simulink model "ModelForSlidesFeb"  (R2023a)
settings: Solver=VariableStepAuto  StartTime=0  StopTime=1000  FixedStep=0.01  RelTol=1e-3
model workspace (MAT data in the model file):
  finalint = 0
  firstWarning = 1
  originalScenarioChecksum = '114339432DE22364D47BB28FC96DC10C'
undefined symbols (not defined in the file): Acceleration, ActorID, AngularVelocity, curvature, DefaultGear, Defined, DEND_B, DEND_S, DEND_T, direction, DiscIntNeverNeededParam, driving, Ego, gradbp, L, Lane, LF, LR, m, matlabshared, MAX_BRAKE, MAX_STEER, MAX_TORQUE, maxNumActors, MCAR, MIN_BRAKE, MIN_STEER, MIN_TORQUE, n, NUMD_B, NUMD_S, NUMD_T, Pitch, Pose, Position, psi_o, R, Roll, RRdamp, SceneInfo, session, sigbuilder_block, STEER_RATIO, stopSign_ID, Tdead, thetaRefs, TL_ID, TrackWidth, ts, Ts, User, Vdead, Velocity, WB, X_o, xRef2s, Y_o, Yaw, yRef2s
libraries: drivingscenarioandsensors x13, roadrunnerscenario x11, simulink x8, simulink_extras x5, drivingvehiclecontroller x2, trackingutilitieslib x2, robotalgslib x1, mpcadaslib x1, slpidlib x1, drivinglib x1, autolibshared x1, vehdynlibviscommon x1
(part 4 of 4)

== matlab function ModelForSlidesFeb/Subsystem/Function-Call Subsystem/MATLAB Function2 ==
  data: EgoPosition input; MIOPos input; curvature input; MIOVel input; V_i input; xd output; yd output; laneL input; laneR input; V_desired input; LCinProgress output
function [xd,yd,LCinProgress] = traj(EgoPosition,MIOPos,curvature,MIOVel, V_i, laneL, laneR, V_desired)
Vx_i =0;Vx_f=0;Vy_i=0;Vy_f=0;Ax_i=0;Ax_f=0;Ay_i=0;Ay_f=0;T_i=0;T_f=0;V_f=0;A_f=0;x_set=0;y_set=0;theta4=0;

P = zeros(6,6);
% xq = zeros(1,size(RefPath,1)); yq = zeros(1,size(RefPath,2));
EgoPosition(1,2)=-EgoPosition(1,2)
x_init= EgoPosition(1,1)+0.5; y_init = EgoPosition(1,2)-0.8;
% xq = RefPath(:,1)'; 
% yq = RefPath(:,2)';
num_foc_t = 98;
V_max= V_desired; ad_n=0; vd_n=MIOVel; wd_n=vd_n*curvature;
lane_width = 3.6 * (laneL-laneR); % +1 if left of current lane and -1 if right of current lane
xd = zeros(num_foc_t+1,1); 
yd = zeros(num_foc_t+1,1);
xf =0; 
yf = 0;

    %xf = [EgoPosition(1,1)+ MIOPos(1) ]; yf = [ EgoPosition(1,2)+ MIOPos(2) + lane_width];  
    xf = [EgoPosition(1,1)+ 40 ]; yf = [ EgoPosition(1,2)+ 1.1*lane_width]; % 80
    V_f = V_max;
    W_f = V_f*curvature;
    A_f = 0;

    %dist2crash = sqrt((x_init-MIOPos(1))^2+(y_init-MIOPos(2))^2);
    %dist2crash = 40;
    %T_f = abs(dist2crash/(MIOVel-V_i));
    T_f = 3;
    P = [1, T_i, T_i^2, T_i^3, T_i^4, T_i^5;
         0, 1, 2*T_i, 3*T_i^2, 4*T_i^3, 5*T_i^4;
         0, 0, 2, 6*T_i, 12*T_i^2, 20*T_i^3;
         1, T_f, T_f^2, T_f^3, T_f^4, T_f^5;
         0, 1, 2*T_f, 3*T_f^2, 4*T_f^3, 5*T_f^4;
         0, 0, 2, 6*T_f, 12*T_f^2, 20*T_f^3];

%     mtang4 = (yq(1,index+2)-yq(1,index+1))/(xq(1,index+2)-xq(1,index+1));

    Vx_i = vd_n*cos(theta4); 
    Vy_i = vd_n*sin(theta4); 
    Ax_i = ad_n*cos(theta4)-vd_n*sin(theta4)*wd_n; 
    Ay_i = ad_n*sin(theta4)+vd_n*cos(theta4)*wd_n;

%     if(xq(index+2)-xq(index+1)<0)
%         theta_4 = pi + atan(mtang4);
%     else
%         theta_4 = atan(mtang4);
%     end

    theta_4 =0;
    Vx_f = V_f*cos(theta_4); % curvature angle
    Vy_f = V_f*sin(theta_4);
    Ax_f = A_f*cos(theta_4)-V_f*sin(theta_4)*W_f;
    Ay_f = A_f*sin(theta_4)+V_f*cos(theta_4)*W_f;

    g1 = [x_init; Vx_i; Ax_i; xf; Vx_f; Ax_f];
    g2 = [y_init; Vy_i; Ay_i; yf; Vy_f; Ay_f];

    a_coeff = P\g1;
    b_coeff = P\g2;
    
    td = T_i;
    scatter(x_init,y_init,'go')
    hold on; 
    scatter(xf,yf,'ro')
    hold on;
    
    for f = 1:(num_foc_t+1)
        xd(f,1) = [1,td,td^2,td^3,td^4,td^5]*a_coeff 
        yd(f,1) = [1,td,td^2,td^3,td^4,td^5]*b_coeff
        td = td + (T_f - T_i)/num_foc_t;
        scatter(xd(f,1),yd(f,1),'y.');
    end

LCinProgress = 1;

% hold on;
end

== matlab function ModelForSlidesFeb/Controllers/MATLAB Function2 ==
  data: v input; RefVelCmd output; curvature input
function RefVelCmd = fcn(v,curvature)

    if abs(curvature) >= 0 && abs(curvature) <= 2e-2
        RefVelCmd = v;
    else
        r = 1/abs(curvature);
        RefVelCmd = min(v,sqrt(9.81*r*.2));
    end

== matlab function ModelForSlidesFeb/Vehicle Dynamics/Info2ActorState/MATLAB Function1 ==
  data: Xdot input; Velocity output; Ydot input; Zdot input
function Velocity = fcn(Xdot, Ydot, Zdot)

Velocity = [Xdot Ydot, Zdot];

== matlab function ModelForSlidesFeb/MATLAB Function ==
  data: ttc output; dist output; left output; right output; LL_avail output; RL_avail output; tend2stay output; ego input; act input; LaneBounds input; RoadSpeed input; ego_vel output; stay output; LL_Change output; RL_Change output; y_lane output; LCinProgress input
function [ttc,dist,left,right,LL_avail,RL_avail,tend2stay,ego_vel,stay,LL_Change,RL_Change,y_lane] = fcn(ego,act,LaneBounds,RoadSpeed, LCinProgress)                       


%% Major tasks to look into

% Check the performance while transitioning into another lane 
% Lane change output when the ego on extreme lanes.
% Develop code to handle lane changes on road curvatures
% Integrate with the trajectory generation and check the perfomance
% Convert the code to ego vehicle coordinates


%%
%define some parameters
r_c = 20; %range considered to MIOs
t_min =  2;

num_actors = length(act.Actors);
%num_lanes = length(LaneBounds.LaneBoundaries)-1;


%% Using sensor data 
% TracksNum = Tracking.NumTracks;
% 
% 
% for t = 1:TracksNum
%     ObjectID(t) = Tracking.Tracks(t).ObjectClassID;
%     TrackPos(:,t) = Tracking.Tracks(t).State(1:2:5);
%     TrackVel(:,t) = Tracking.Tracks(t).State(2:2:6);

%% ego position and  velocity magnitude
ego_pos = ego.Position;
ego_vel = ego.Velocity(1);  % velocity

%ttc: (array) : agent.relative position / abs(relative velocity)
ttc = zeros(1,num_actors);
left = zeros(1,num_actors);
right = zeros(1,num_actors);

dist =  zeros(1,num_actors);
tend2stay=1;

%%
y_lane = zeros(1,length(LaneBounds.LaneBoundaries))

for l=1:length(y_lane)
    y_lane(l)=LaneBounds.LaneBoundaries(l).Coordinates(end,2)
end

%%
for i= 1:num_actors

    % Grab actor positions and velocities
    actor_pos = act.Actors(i).Position;   
    actor_vel = act.Actors(i).Velocity(1);  % x-component velocity

    %relative velocity of the agent
    rel_vel = actor_vel - ego_vel;


    %% Check if the actor is within a r_c range. If it is out of range, pass lane change as '1' automatically.

   dist(i) = norm([actor_pos(1) actor_pos(2)]-[ego_pos(1) ego_pos(2)]);
        
    if dist(i) > r_c
        left(i)=1;
        right(i)=1;
        continue
    end

    %% Check if the actor is in the same lane as that of ego

    % If the actor and ego are in the same lane, it is considered a lead/following vehicle in the same lane and by defualt, the lane change flag is 1.

    if (actor_pos(2)< (ego_pos(2)+0.5) && actor_pos(2) > (ego_pos(2)-0.5))
        if (rel_vel < 0 && ego_vel < (RoadSpeed+5) && actor_pos(1) > ego_pos(1) )
            left(i) =1;
            right(i)=1;
            tend2stay=0;        % we need to incorporate too slow condition even when the relative velocity is greater than 0.

        elseif (rel_vel < 0 && ego_vel < (RoadSpeed+5) && actor_pos(1) < ego_pos(1) )
            left(i) =1;
            right(i)=1;
            tend2stay=1;
        end

        continue
    end

    
    %% calculate ttc for the rest of the vehicles


    ttc(i) = (actor_pos(1)-ego_pos(1))/abs(rel_vel);

    % checking conditions for other surrounding actors

    % all actors on the left lane of the ego vehicle
%%
    if actor_pos(2)-ego_pos(2) > 0  

        if and(rel_vel>0, ttc(i) > t_min)  % target vehicles on the front of ego vehicle (any lane)
    
            left(i)=1; 
            right(i)=1;
    
        elseif (ttc(i)<0 && rel_vel<0 && abs(ttc(i)) > t_min)    % target vehicle on the back of ego vehicle (ttc<0) (any lane)
            left(i) =1;
            right(i)=1;
    
        else 
            left(i) =0;
            right(i)=1;
    
        end

    % all actors on the right lane of the ego vehicle

    elseif actor_pos(2)-ego_pos(2) < 0
         
        if and(rel_vel>0, ttc(i) > t_min)  % target vehicles on the front of ego vehicle (any lane)
    
            left(i)=1;
            right(i)=1;
    
        elseif (ttc(i)<0 && rel_vel<0 && abs(ttc(i)) > t_min)    % target vehicle on the back of ego vehicle (ttc<0) (any lane)
            left(i) =1;
            right(i)=1;
    
        else 
            left(i) =1;
            right(i)=0;
    
        end
    end
%%

end

%% check if the vehicle is in the extreme end lanes

    if ego_pos(2)<y_lane(1) && ego_pos(2)>y_lane(2)

        LL=0; RL=1;
    elseif ego_pos(2) > y_lane(end) && ego_pos(2) < y_lane(end-1)
        RL=0; LL=1;
    else 

        RL=1;LL=1;
    end

%%
LL_avail = all(left) %&& LL;

RL_avail = all(right) %&& RL               %&& ~lcLeft ; this can be decided later 


%% final commands

stay = tend2stay || ~(tend2stay || LL_avail || RL_avail);
LL_Change =  ~tend2stay && LL_avail ;

RL_Change =  ~tend2stay && RL_avail && ~LL_Change ;
LCFlag = ~stay;
if LCFlag && LCinProgress
    LCFlag = false;
    stay = ~LCFlag;
end

%% 






end

== matlab function ModelForSlidesFeb/Vehicle Dynamics/Info2ActorState/MATLAB Function2 ==
  data: aX input; Acceleration output; aY input; aZ input
function Acceleration = fcn(aX, aY, aZ)

Acceleration = [aX aY, aZ];

== matlab function ModelForSlidesFeb/Vehicle Dynamics/Info2ActorState/MATLAB Function3 ==
  data: phiDot input; AngularVelocity output; thetaDot input; psiDot input
function AngularVelocity = fcn(phiDot, thetaDot, psiDot)

AngularVelocity = [phiDot thetaDot, psiDot];

== stateflow chart ModelForSlidesFeb/Vehicle Dynamics/VehicleDynamics/engine-steer-brake dynamics/GearSelection1 ==
  state Park
    CurrGear = 0;
  state Reverse
    CurrGear = -1;
  state drive
    CurrGear = 1;
  (default) -> (junction 12)
  (junction 12) -> Reverse [order 3] : [DefaultGear == -1]
  (junction 12) -> drive [order 2] : [DefaultGear == 1]
  (junction 12) -> Park [order 1] : [DefaultGear == 0]
  (junction 12) -> Park [order 4] : %fallback to park
  drive -> Park [order 2] : [gear_cmd == 0 && allowShift(vc,Tbrake)]
  Park -> Reverse [order 2] : [gear_cmd == -1 && allowShift(vc,Tbrake)]
  Park -> drive [order 1] : [gear_cmd == 1 && allowShift(vc,Tbrake)]
  Reverse -> Park [order 2] : [gear_cmd == 0 && allowShift(vc,Tbrake)]
  drive -> Reverse [order 1] : [gear_cmd == -1 && allowShift(vc,Tbrake)]
  Reverse -> drive [order 1] : [gear_cmd == 1 && allowShift(vc,Tbrake)]
  data: Tdead parameter; Vdead parameter; vel function_input; brakeT function_input; allow function_output; CurrGear output; Tbrake input; vc input; gear_cmd input; DefaultGear parameter
  function allow = allowShift(vel, brakeT):
    | function allow = allowShift(vel, brakeT)
    | allow = (abs(vel) <= Vdead) && (abs(brakeT)>Tdead);
    | end

== matlab function ModelForSlidesFeb/Vehicle Dynamics/VehicleDynamics/engine-steer-brake dynamics/compute net torque ==
  data: gear input; Tnet output; Tengine input; Tbrake input; vc input
function Tnet  = net_torque(gear,Tengine,Tbrake,vc)

%  --set engine torque based on current gear selection

if (gear == 0)
    %  --vehicle is in PARK, so force engine torque to zero
    Tengine = 0;
end

Tnet = Tengine + Tbrake*tanh(5*vc);

end

== matlab function ModelForSlidesFeb/Vehicle Dynamics/VehicleDynamics/engine-steer-brake dynamics/gear selection state machine ==
  data: gear output; gear_cmd input; vc input; Tbrake input; Tdead input; Vdead input
function gear = gear_change_FSM(gear_cmd,vc,Tbrake,Tdead,Vdead)

persistent GEAR

%  The vehicle gear can take on one of the following enumerated values:
%  -1 = REVERSE
%   0 = PARK
%   1 = DRIVE

%  --initialize the local persistent variables

if isempty(GEAR)
    %  --default gear at startup is PARK
    %  Note:  Change this to 1 if you want car to initialize in DRIVE
    GEAR = 0;
end


%  --evaluate the gear change finite state machine

switch GEAR
    case 0  % vehicle is in PARK
        if (gear_cmd == 1)
            %  --check to see if we can shift to DRIVE
            if ((abs(vc) <= Vdead) && (abs(Tbrake) > Tdead))
                %  --shift to DRIVE
                GEAR = 1;
            end
            
        elseif (gear_cmd == 2)
            %  --check to see if we can shift to REVERSE
            if ((abs(vc) <= Vdead) && (abs(Tbrake) > Tdead))
                %  --shift to REVERSE
                GEAR = 2;
            end
        end
        
    case 1  % vehicle is in DRIVE
        if (gear_cmd == 0)
            %  --check to see if we can shift to PARK
            if ((abs(vc) <= Vdead) && (abs(Tbrake) > Tdead))
                %  --shift to PARK
                GEAR = 0;
            end
            
        elseif (gear_cmd == 2)
            %  --check to see if we can shift to REVERSE
            if ((abs(vc) <= Vdead) && (abs(Tbrake) > Tdead))
                %  --shift to REVERSE
                GEAR = 2;
            end
        end
        
    case -1  % vehicle is in REVERSE
        if (gear_cmd == 0)
            %  --check to see if we can shift to PARK
            if ((abs(vc) <= Vdead) && (abs(Tbrake) > Tdead))
                %  --shift to PARK
                GEAR = 0;
            end
            
        elseif (gear_cmd == 1)
            %  --check to see if we can shift to DRIVE
            if ((abs(vc) <= Vdead) && (abs(Tbrake) > Tdead))
                %  --shift to DRIVE
                GEAR = 1;
            end
        end
        
    otherwise  %  --should never be here
        if (vc > Vdead)
            %  --moving forward, so must be in DRIVE
            GEAR = 1;
        elseif (vc < -Vdead)
            %  --moving backward, so must be in REVERSE
            GEAR = 2;
        else
            %  --vehicle stoppped, so must be in PARK
            GEAR = 0;
        end

end


%  --output the current actual gear setting

gear = GEAR;

return

== matlab function ModelForSlidesFeb/Behavioural Planner/MATLAB Function3 ==
  data: Dest input; D2D output; CurrentPose input
function D2D = fcn(Dest, CurrentPose)

% CurrentPose(2) = -CurrentPose(2);

% For RoadRunner
Dest = [Dest(2) Dest(1)]; 
CurrentPose = [CurrentPose(2) CurrentPose(1)];
D2D = norm(Dest - CurrentPose(1:2));

% D2D=sqrt((CurrentPose(1)-Dest(1,1))^2+(CurrentPose(2)-Dest(1,2))^2);
end

== stateflow chart ModelForSlidesFeb/Behavioural Planner/Chart ==
  settings: updateMethod=DISCRETE  sampleTime=Ts
  state Stationary
    en,du:
    VelCmd = 0;
    CurrentVelCmd = VelCmd;
    Navi = 0;
    Trans = 0;
    StopSim = 0;
    Tgap = 1;
    HoldBrake = 1;
    Braking = 0;
  state Navigation
    state RailCrossing
      state Stop
        en:
        VelCmd = 0;
        Braking = 1;
        CurrentVelCmd = VelCmd;
      state Approaching
        en:
        Braking = 1;
        Tgap = 0;
        Trans = 0;
      state Transition
        en:
        Tgap = 1;
        Trans = 1;
        Braking = 0;
        VelCmd = SceneSpeed;
        CurrentVelCmd = VelCmd;
      state ExitScene
        en:
        ExitFlag = 1;
      (default) -> Navigation.RailCrossing.Approaching
      Navigation.RailCrossing.Approaching -> Navigation.RailCrossing.Stop [order 1] : [D2S <= 6 && (RRCross == 1 || ObjectDist <= TransDist)]
      Navigation.RailCrossing.Transition -> Navigation.RailCrossing.Approaching [order 2] : [ObjectDist <= TransDist]
      Navigation.RailCrossing.Approaching -> Navigation.RailCrossing.Transition [order 3] : [RRCross == 0 && ObjectDist > TransDist && D2S <= 6]
      Navigation.RailCrossing.Stop -> Navigation.RailCrossing.Transition : [RRCross == 0 && ObjectDist > TransDist]
      Navigation.RailCrossing.Approaching -> Navigation.RailCrossing.ExitScene [order 2] : [SceneID ~= 10]
      Navigation.RailCrossing.Transition -> Navigation.RailCrossing.ExitScene [order 1] : [SceneID == 0]
    state RoundAbout
      state Approaching
        en:
        Braking = 1;
        Trans = 0;
        Tgap = 0;
      state Stop
        en:
        VelCmd = 0;
        Braking = 1;
        CurrentVelCmd = VelCmd;
      state ExitScene
        en:
        ExitFlag = 1;
      state Transition
        en:
        Tgap = 1;
        Trans = 1;
        Braking = 0;
        VelCmd = SceneSpeed;
        CurrentVelCmd = VelCmd;
      (default) -> Navigation.RoundAbout.Approaching
      Navigation.RoundAbout.Approaching -> Navigation.RoundAbout.Stop [order 1] : [D2S <= 6]
      Navigation.RoundAbout.Stop -> Navigation.RoundAbout.Transition : [Clear2Go == 1]
      Navigation.RoundAbout.Approaching -> Navigation.RoundAbout.ExitScene [order 2] : [SceneID ~= 9]
      Navigation.RoundAbout.Transition -> Navigation.RoundAbout.ExitScene : [SceneID == 0]
    state DestCheck
      en,du:
      % dest reached?
      (default) -> (junction 47)
      (junction 47) -> (junction 48) [order 1] : [D2D < 2]
      (junction 47) -> (junction 49) [order 2] : {DestReached = 0;}
      (junction 48) -> (junction 50) : {DestReached = 1;}
      (junction 50) -> (junction 49) : {StopSim = 1;}
      (junction 49) -> (junction 51)
    state TrafficLight [commented out]
      note: Yellow light duration is 1s
      state Stop [commented out]
        en:
        Braking = 1;
        VelCmd = 0;
        CurrentVelCmd = VelCmd;
      state Approaching [commented out]
        en:
        Tgap = 0;
        Trans = 0;
        T2S = 0;
        %if TLstate(1,4) == 1
        Braking = 1;
        %else
        % ACC = 0;
        %end
      state DecisionOnYellow [commented out]
        en:
        T2S = D2S/EgoSpeed;
      state Transition [commented out]
        en:
        Trans = 1;
        Braking = 0;
        Tgap = 1;
        VelCmd = SceneSpeed;
        CurrentVelCmd = VelCmd;
      state ExitScene [commented out]
        en:
        ExitFlag = 1;
      DecisionOnYellow -> Navigation.TrafficLight.Approaching [commented out] : [T2S > 1.2]
      (default) -> Navigation.TrafficLight.Approaching [commented out]
      Navigation.TrafficLight.Approaching -> Navigation.TrafficLight.Stop [commented out] : [D2S <= 6]
      Navigation.TrafficLight.Stop -> Navigation.TrafficLight.Transition [commented out] : [TLstate(1,4) == 3 && ObjectDist > TransDist]
      Navigation.TrafficLight.Transition -> Navigation.TrafficLight.Approaching [commented out] : [TLstate(1,4) == 1  || ObjectDist < TransDist]
      Navigation.TrafficLight.Approaching -> Navigation.TrafficLight.Transition [commented out] : [TLstate(1,4) == 3 && ObjectDist > TransDist]
      Navigation.TrafficLight.Approaching -> Navigation.TrafficLight.ExitScene [commented out] : [SceneID ~= 8]
      Navigation.TrafficLight.Transition -> DecisionOnYellow [commented out] : [TLstate(1,4) == 2]
      DecisionOnYellow -> Navigation.TrafficLight.Transition [commented out] : [T2S <= 1.2]
      Navigation.TrafficLight.Transition -> Navigation.TrafficLight.ExitScene [commented out] : [SceneID == 0]
    state Drive
      en :
      HoldBrake = 0;
      VelCmd = RoadSpeed;
      CurrentVelCmd = VelCmd;
      ExitFlag = 0;
    state Go
      en:
      VelCmd = RoadSpeed;
      CurrentVelCmd = VelCmd;
      Trans = 0;
      ExitFlag = 0;
      Braking = 0;
      HoldBrake = 1;
    state StopSign
      state StoptSign4way
        state CheckInt
          du:
          % stopped?
          % ss priority?
        state CheckSS
          % stopped?
          % ss priority?
        state Transition
          en:
          % stay here while trans?!
          % while ~crossedLimitLine of TargetLane
          Trans = 1;
          Braking = 0;
          Tgap = 1;
          VelCmd = SceneSpeed;
          CurrentVelCmd = VelCmd;
        state ExitScene
          en:
          ExitFlag = 1;
        (default) -> Navigation.StopSign.StoptSign4way.CheckSS
        Navigation.StopSign.StoptSign4way.CheckSS -> Navigation.StopSign.StoptSign4way.CheckInt : [EgoSpeed < VelStop]
        Navigation.StopSign.StoptSign4way.CheckInt -> Navigation.StopSign.StoptSign4way.Transition : [egoSSPriority == 1 && Clear2Go == 1]
        Navigation.StopSign.StoptSign4way.Transition -> Navigation.StopSign.StoptSign4way.ExitScene : [SceneID == 0 && after(2,sec)]
      state SStype
        state Approaching
          en:
          %VelCmd = ApproachingSpeed;
          Braking = 1;
          Trans = 0;
          Tgap = 0;
        state Stop
          en:
          VelCmd = 0;
          Braking = 1;
          CurrentVelCmd = VelCmd;
        Navigation.StopSign.SStype.Stop -> 410 [order 1] : [numSS == 4]
        (default) -> Navigation.StopSign.SStype.Approaching
        Navigation.StopSign.SStype.Approaching -> Navigation.StopSign.SStype.Stop : [D2S <= 15]
        Navigation.StopSign.SStype.Stop -> 414 [order 2] : [numSS == 2]
      state StopSign2way
        state CheckInt
          en:
          VelCmd = 0;
          HoldBrake = 1;
          CurrentVelCmd = VelCmd;
        state CheckSS
          % stopped?
          % ss priority?
        state Transition1
          en:
          % stay here while trans?!
          % while ~crossedLimitLine of TargetLane
          Trans = 1;
          Braking = 0;
          HoldBrake = 0;
          Tgap = 1;
          VelCmd = SceneSpeed;
          CurrentVelCmd = VelCmd;
        state ExitScene1
          en:
          ExitFlag = 1;
        (default) -> Navigation.StopSign.StopSign2way.CheckSS
        Navigation.StopSign.StopSign2way.CheckSS -> Navigation.StopSign.StopSign2way.CheckInt : [EgoSpeed < VelStop]
        Navigation.StopSign.StopSign2way.CheckInt -> Transition1 : [egoSSPriority == 1 && ToAClearance == 1 && after(1,sec)]
        Transition1 -> Navigation.StopSign.StopSign2way.CheckInt [order 2] : [ToAClearance == 0]
        Transition1 -> ExitScene1 [order 1] : [SceneID == 0 && egoExit == 1]
      (default) -> SStype
      416 -> StoptSign4way
      411 -> StopSign2way
    Go -> RailCrossing [order 2] : [SceneID == 10]
    Drive -> RailCrossing [order 1] : [SceneID == 10]
    RailCrossing -> Go : [ExitFlag == 1]
    Go -> RoundAbout [order 3] : [SceneID == 9]
    Drive -> RoundAbout [order 2] : [SceneID == 9]
    RoundAbout -> Go : [ExitFlag == 1]
    (default) -> DestCheck
    Drive -> TrafficLight [commented out] : [SceneID == 8]
    DestCheck -> Drive : [DestReached == 0]
    Go -> TrafficLight [commented out] : [SceneID == 8]
    Drive -> DestCheck [order 4] : [D2D < 2]
    TrafficLight -> Go [commented out] : [ExitFlag == 1]
    Drive -> StopSign [order 3] : [SceneID == 7]
    StopSign -> Go : [ExitFlag == 1]
    Go -> DestCheck [order 1] : [SceneID == 0]
    Go -> StopSign [order 4] : [SceneID == 7]
  (default) -> Stationary
  Stationary -> Navigation : [Navigate == 1]
  Navigation -> Stationary : [Navigate == 0 || DestReached == 1]
  data: TLstate input; numSS input; egoExit input; ToAClearance input; TransDist input; ApproachingSpeed input; EgoSpeed input; ObjectDist input; SceneSpeed input; SDist input; RRCross input; D2S input; DestReached local; Navigate input; ExitFlag local; D2D input; Clear2Go input; RoadSpeed input; CurrentVelCmd local; Navi local; VelCmd output; HoldBrake output; SceneID input; Tgap output; Trans output; StopSim output; Braking output; T2S local; VelStop input; egoSSPriority input

== matlab function ModelForSlidesFeb/Subsystem/Function-Call Subsystem/MATLAB Function1 ==
  data: EgoPosition input; MIOPos input; curvature input; MIOVel input; V_i input; xd output; yd output; laneL input; laneR input; V_desired input; LCinProgress output
function [xd,yd,LCinProgress] = traj(EgoPosition,MIOPos,curvature,MIOVel, V_i, laneL, laneR, V_desired)
Vx_i =0;Vx_f=0;Vy_i=0;Vy_f=0;Ax_i=0;Ax_f=0;Ay_i=0;Ay_f=0;T_i=0;T_f=0;V_f=0;A_f=0;x_set=0;y_set=0;theta4=0;

P = zeros(6,6);
% xq = zeros(1,size(RefPath,1)); yq = zeros(1,size(RefPath,2));
EgoPosition(1,2)=-EgoPosition(1,2);
x_init= EgoPosition(1,1)+2; y_init = EgoPosition(1,2)-2;
% xq = RefPath(:,1)'; 
% yq = RefPath(:,2)';
num_foc_t = 98;
V_max= V_desired; ad_n=0; vd_n=MIOVel; wd_n=vd_n*curvature;
lane_width = 3.6 * (laneL-laneR); % +1 if left of current lane and -1 if right of current lane(rahul flipped)
xd = zeros(num_foc_t+1,1); 
yd = zeros(num_foc_t+1,1);
xf =0; 
yf = 0;

    %xf = [EgoPosition(1,1)+ MIOPos(1) ]; yf = [ EgoPosition(1,2)+ MIOPos(2) + lane_width];  
    xf = [EgoPosition(1,1)+ 20 ]; yf = [EgoPosition(1,2)+ lane_width]; % 80
    V_f = V_max;
    W_f = V_f*curvature;
    A_f = 0;

    %dist2crash = sqrt((x_init-MIOPos(1))^2+(y_init-MIOPos(2))^2);
    %dist2crash = 40;
    %T_f = abs(dist2crash/(MIOVel-V_i));
    T_f = 3;
    P = [1, T_i, T_i^2, T_i^3, T_i^4, T_i^5;
         0, 1, 2*T_i, 3*T_i^2, 4*T_i^3, 5*T_i^4;
         0, 0, 2, 6*T_i, 12*T_i^2, 20*T_i^3;
         1, T_f, T_f^2, T_f^3, T_f^4, T_f^5;
         0, 1, 2*T_f, 3*T_f^2, 4*T_f^3, 5*T_f^4;
         0, 0, 2, 6*T_f, 12*T_f^2, 20*T_f^3];

%     mtang4 = (yq(1,index+2)-yq(1,index+1))/(xq(1,index+2)-xq(1,index+1));

    Vx_i = vd_n*cos(theta4); 
    Vy_i = vd_n*sin(theta4); 
    Ax_i = ad_n*cos(theta4)-vd_n*sin(theta4)*wd_n; 
    Ay_i = ad_n*sin(theta4)+vd_n*cos(theta4)*wd_n;

%     if(xq(index+2)-xq(index+1)<0)
%         theta_4 = pi + atan(mtang4);
%     else
%         theta_4 = atan(mtang4);
%     end

    theta_4 =0;
    Vx_f = V_f*cos(theta_4); % curvature angle
    Vy_f = V_f*sin(theta_4);
    Ax_f = A_f*cos(theta_4)-V_f*sin(theta_4)*W_f;
    Ay_f = A_f*sin(theta_4)+V_f*cos(theta_4)*W_f;

    g1 = [x_init; Vx_i; Ax_i; xf; Vx_f; Ax_f];
    g2 = [y_init; Vy_i; Ay_i; yf; Vy_f; Ay_f];

    a_coeff = P\g1;
    b_coeff = P\g2;
    
    td = T_i;
    scatter(x_init,y_init,'go')
    hold on; 
    scatter(xf,yf,'ro')
    hold on;
    
    for f = 1:(num_foc_t+1)
        xd(f,1) = [1,td,td^2,td^3,td^4,td^5]*a_coeff 
        yd(f,1) = [1,td,td^2,td^3,td^4,td^5]*b_coeff
        td = td + (T_f - T_i)/num_foc_t;
        scatter(xd(f,1),yd(f,1),'y.');
    end

LCinProgress = 1;

% hold on;
end

== matlab function ModelForSlidesFeb/Behavioural Planner/StopSignPriority ==
  settings: updateMethod=DISCRETE
  data: ToAClearance output; SDist input; D2S input; ObjTracks input; egoSSPriority output; SceneTracks input; egoPose input; egoSpeed input; numSS output; VelStop input; WB input; d output; flag input; flag output; midpoint input; midpoint output; egoExit output; egoEnter input; egoEnter output; egoExitang output; egoExitdist output
function [ToAClearance, egoSSPriority, numSS, d, flag, midpoint, egoExit, egoEnter, egoExitang, egoExitdist]  = StopSignPriority(SDist, D2S, ObjTracks, SceneTracks, egoPose, egoSpeed, VelStop, WB, flag, midpoint, egoEnter)
% calculate covariance matrix outside, input to this block is modified with final, unique detections
egoPose = [-egoPose(2) egoPose(1) 90+egoPose(3)];
persistent SSPriority C1x C2y C3x C4y
% find stop signs + one of 2way or 4way or T-junction

% find number of signs (until we reach 0 valued columns)
numSS = 0;
for j = 1:length(SceneTracks(1,:))
    if any(SceneTracks(:,j))
        numSS = numSS + 1;
    end
end

% find number of cars
numCars = 0;
for j = 1:length(ObjTracks(1,:))
    if any(ObjTracks(:,j))
        numCars = numCars + 1;
    end
end


egoSSPriority = 1;
ToAClearance = 1;
actorExitang = 0;
ToAThreshold = 5;
% tempPriority = zeros(numCars+1,1);
d = zeros(10, 5); % distance, velocity, time, location (wrt ego), exit (leaving ints)
Objang = zeros(10, 1);
% priorityTable = zeros(numCars+1, 5);
egoExitang = egoPose(3) - atan2d(midpoint(2)-egoPose(2),midpoint(1)-egoPose(1)); % 0 deg = straight , + = right
egoExitdist = sqrt((midpoint(2)-egoPose(2))^2+(midpoint(1)-egoPose(1))^2);

if abs(egoExitang) >= 135 && egoExitdist >= 10 && egoEnter == 1
    d(1,5) = 1; % ego left the ints
    egoEnter = 0;
    flag = 0;
elseif abs(egoExitang) >= 135 && egoExitdist <= 20 && egoExitdist >= 10
    d(1,5) = 1;
end

egoExit = d(1,5);


if (D2S <= SDist || egoEnter == 1) && egoExitdist >= 9

    % [~, index] = min(abs(SceneTracks(1,:)'));
    if numSS > 0

        Vmd = [-egoSpeed*sind(egoPose(3)), egoSpeed*cosd(egoPose(3))];
        rot = [cosd(egoPose(3)) -sind(egoPose(3)); sind(egoPose(3)) cosd(egoPose(3))];
        

        % intersection region
        if flag == 0
            C1x = min(SceneTracks(1, 1:numSS)) - (WB + 3);
            C2y = min(SceneTracks(3, 1:numSS)) - (WB + 3);
            C3x = max(SceneTracks(1, 1:numSS)) + (WB + 3);
            C4y = max(SceneTracks(3, 1:numSS)) + (WB + 3);
            C1 = rot*[C1x; C2y] + egoPose(1:2)';
            C2 = rot*[C3x; C4y] + egoPose(1:2)';
            midpoint = (C1+C2)./2;
            
            % C1x = min(SceneTracks(1, 1:numSS)) - (WB + 3);
            % C2y = min(SceneTracks(3, 1:numSS)) - (WB + 3);
            % C3x = max(SceneTracks(1, 1:numSS)) + (WB + 3);
            % C4y = max(SceneTracks(3, 1:numSS)) + (WB + 3);
            % midpoint = [2*egoPose(1)-C4y-C2y; 2*egoPose(2)+C1x+C3x]./2;
        %   scatter(-SceneTracks(3,:)+egoPose(1),SceneTracks(1,:)+egoPose(2),'blue','filled')   
            % scatter(midpoint(1), midpoint(2), 'blue', 'filled')
            % rectangle('Position',[egoPose(1)-C4y egoPose(2)+C1x abs(C4y-C2y) abs(C3x-C1x)])
            flag = C1x;
        end

        midpoint_ego = rot'*(midpoint - egoPose(1:2)');
        
        % loop through num of cars (j)
    
        d(1,1) = sqrt((midpoint(1) - egoPose(1))^2 + (midpoint(2) - egoPose(2))^2);
        d(1,2) = egoSpeed;
        d(1,3) = d(1,1)/d(1,2);     %add ego TOA
        d(1,4) = 4; % 4 is the location of the ego vehicle itself
        
        % if d(1,1) <= 3
        %     ToAThreshold = 2;
        % else
        %     ToAThreshold = 6;
        % end

        if d(1,1) <= flag
            egoEnter = 1;
        end

    
        % loop through signs (vectorized)
        % if smallest dist 
        % d(:,3) -> TOA = v/dist
    
        if numCars > 0
            for k = 1:numCars
                d(k+1,1) = sqrt((midpoint_ego(2)-ObjTracks(3,k))^2+(midpoint_ego(1)-ObjTracks(1,k))^2); %sqrt((midpoint(1) - (-ObjTracks(3,k)+egoPose(1)))^2 + (midpoint(2) - (ObjTracks(1,k)+egoPose(2)))^2); 
                d(k+1,2) = sqrt((Vmd(1) - ObjTracks(2,k))^2 + (Vmd(2) - ObjTracks(4,k))^2);
                d(k+1,3) = d(k+1,1)/d(k+1,2); % TOA of other cars
                Objang(k) = atan2d(ObjTracks(1,k), -ObjTracks(3,k));
                                
                % Identify cars location (direction) wrt ego
                if Objang(k) <= 60
                    d(k+1,4) = 1; % 1 = E, 2 = N, 3 = W
                elseif Objang(k) > 60  && Objang(k) < 120
                    d(k+1,4) = 2; % 1 = E, 2 = N, 3 = W
                elseif Objang(k) >= 120
                    d(k+1,4) = 3; % 1 = E, 2 = N, 3 = W
                end

                % Identifying leaving cars
                
                % ActorHeading = atan2d(ObjTracks(2,k) - Vmd(1), -ObjTracks(4,k) - Vmd(2));
                ActorHeading = atan2d(ObjTracks(2,k), ObjTracks(4,k));
                actorExitTheta = ActorHeading - atan2d(midpoint_ego(1)-ObjTracks(1,k),midpoint_ego(2)-ObjTracks(3,k));
                if actorExitTheta > 180
                    actorExitang = actorExitTheta - 360;
                else
                    actorExitang = actorExitTheta;
                end
                %actorExitdist = sqrt((midpoint_ego(2)-ObjTracks(3,k))^2+(midpoint_ego(1)-ObjTracks(1,k))^2);
                

                if abs(actorExitang) >= 135 && d(k+1,1) >= 10 
                    d(k+1,5) = 1; % left the ints
                else
                    d(k+1,5) = 0; % did not leave
                end

    
            end
    
            if numSS == 4 
                % Assign priorities based on rank TOA #1, before vehicle stops
                % d1 = d(d(:,1)~=0,:);
                [car, SSPriority] = sort(d(d(:,1)~=0 & d(:,5)==0));
                % priorityTable(:, 1:2) = [car, priority];
        
                tempPriority = find(SSPriority == 1); % ego SS priority
                if ~isempty(tempPriority)
                    egoSSPriority = tempPriority(1);
                end
            
            elseif numSS >= 1 && numSS < 4
                [car, SSPriority] = sort(d((d(:,4)==2 | d(:,4)==4) & d(:,5)==0));
                tempPriority = find(SSPriority == 1); % ego SS priority
                if ~isempty(tempPriority)
                    egoSSPriority = tempPriority(1);              
                end
                ToAClearance = double(all(d(d(:,1)~=0 & d(:,5)==0 & d(:,4)~=4,3) > ToAThreshold));
                
            end
    
        end
    end
    
    
    
    
    % if egoSpeed <= VelStop
    %     if SSPriority ~= 1
    %         % for all vehicles with higher priority
    %         % provide indicator signals to identify conflicts
    %         % check indicator signs/conflicts and update priority based on that
    %         % code to define leavingScene for other vehicles:
    %         % update priority table
    % 
    %     end
    % end
    
    
    
    

% elseif egoExit == 0
    

end

== matlab function ModelForSlidesFeb/Behavioural Planner/MATLAB Function1 ==
  data: EgoLength input; TransDist output; IntDist input
function TransDist = IntersectionClearanceDist(EgoLength,IntDist)

TransDist = IntDist + EgoLength;

== matlab function ModelForSlidesFeb/Subsystem/Turns LC in prog off ==
  data: u input; y output
function y = fcn(u)

persistent counter;
persistent input_high;

if isempty(counter)
    counter = 0;
end

if isempty(input_high)
    input_high = false;
end

if u ~= 0
    input_high = true;
end

if input_high && counter < 100
    y = u;
    counter = counter + 1;
else
    y = 0;
end

== matlab function ModelForSlidesFeb/Environment & Data/Roadrunner Port/ENU to NWD/MATLAB Function ==
  data: traj input; destination_traj output; last_idx output; Initial_traj output
function [destination_traj,last_idx,Initial_traj] = DestinationPoint(traj)

last_idx = 1;

for i=1:length(traj)
    if norm(traj(i,1:2)) == 0
        last_idx = i-1;
        break
    end
end

destination_traj = traj(last_idx,1:2);
Initial_traj = traj(1,1:2);

end

== matlab function ModelForSlidesFeb/Environment & Data/Roadrunner Port/ENU to NWD/MATLAB Function1 ==
  data: traj input; trajectory_way output
function trajectory_way = fcn(traj)

last_idx = 1;

for i=1:length(traj)
    if norm(traj(i,1:2)) == 0
        last_idx = i-1;
        break
    end
end

trajectory_way = zeros(150,2);

for j = 1:last_idx
    trajectory_way(j,:) = traj(j,1:2);
end


for k = (last_idx+1):100
    trajectory_way(k,:) = trajectory_way(last_idx,:);
end

== matlab function ModelForSlidesFeb/Environment & Data/Roadrunner Port/Initiaal State/Initialize State/Calculate Initial States/Calculate Initial States ==
  data: egoRuntime input; egoInitialState output Bus: BusVehicleInfo
function egoInitialState = getInitialState(egoRuntime)
%getInitialState calculates initial conditions of the vehicle

% Calculate velocity
velocity = norm(egoRuntime.ActorRuntime.Velocity,2);
% Get Transformation matrix
transformationMatrix = egoRuntime.ActorRuntime.Pose;
% Get pose information
x = transformationMatrix(1,4);
y = transformationMatrix(2,4);
yaw = atan2d(-transformationMatrix(1,2), ...
            transformationMatrix(1,1));
% Pack the initial states
egoInitialState = struct('CurrPose', [y, -x, yaw], ...
    'CurrVelocity', velocity, ...
    'CurrYawRate', 0, ...
    'CurrSteer',0, ...
    'Direction',1);

== matlab function ModelForSlidesFeb/Environment & Data/Roadrunner Port/MATLAB Function ==
  data: ActorsIn input; EgoVeh input; EgoRefActors output Bus: BusWorldToVehicleActors
function EgoRefActors  = GlobaltoEgoRefConv(ActorsIn,EgoVeh)
%ActorsOut = Simulink.Bus;
ActorsOut = ActorsIn;
numActors = length(ActorsIn.Actors);
for k = 1:numActors
    actorOut = driving.scenario.targetsToEgo(ActorsIn.Actors(k),EgoVeh);
    ActorsOut.Actors(k).ActorID             = actorOut.ActorID;
    ActorsOut.Actors(k).Position            = actorOut.Position;
    ActorsOut.Actors(k).Velocity            = actorOut.Velocity;
    ActorsOut.Actors(k).Roll                = actorOut.Roll;
    ActorsOut.Actors(k).Pitch               = actorOut.Pitch;
    ActorsOut.Actors(k).Yaw                 = actorOut.Yaw;
    ActorsOut.Actors(k).AngularVelocity    = actorOut.AngularVelocity;
end
EgoRefActors = ActorsOut;
end

== matlab function ModelForSlidesFeb/Subsystem/PathPlanner/MATLAB Function3 ==
  settings: updateMethod=DISCRETE
  data: out output; check output; Xref input; Yref input; xd input; yd input; LC input; current_pos input; d2f input; dcheck output
function [out,check,dcheck]  = PathPlanning(Xref, Yref, xd, yd, LC, current_pos, d2f)

persistent output_matrix
persistent lc_triggered

if isempty(lc_triggered)
lc_triggered = false;
end

%lc_triggered=0;
%if isempty(hold_output)
  %  hold_output = false;
%end


if isempty(output_matrix)
    output_matrix = [Xref(:), Yref(:)];
    out = [Xref(:), Yref(:)];
else
    out = output_matrix;
end

if LC && ~isempty(xd) && ~isempty(yd)
    output_matrix = [xd(:), yd(:)];
    lc_triggered=true;
       
end

check=lc_triggered;
dcheck=output_matrix;
%out=output_matrix;

if lc_triggered && d2f < 5 %&& ~isempty(output_matrix) %&& ~hold_output
    %Yout = Yref(:);
    if current_pos > 0
        Xout = Xref(:);
        Yout = Yref + 3.6;
    else
        Xout = Xref(:);
        Yout = Yref;
    end
    output_matrix = [Xout, Yout];
    out=output_matrix;
    lc_triggered=false;
    %hold_output = true;
end

out=output_matrix;




%if ~LC && ~isempty(output_matrix) && lc_triggered
    %hold_output = false;
    %lc_triggered=false;
%end

end

== matlab function ModelForSlidesFeb/Environment & Data/Roadrunner Port/MATLAB Function1 ==
  data: u input; long_out output; lat_out output; z_out output; out output; final_x output; final_y output
function [long_out, lat_out, z_out, out, final_x, final_y]  = fcn(u)
out = zeros(500, 3);
long = zeros(500, 1);
lat = zeros(500, 1);
long = u(:, 2);
lat = u(:,1);

for i = 1:500
    if long(i) == 0 && lat(i) == 0
        long(i) = long(i-1); 
        lat(i) = lat(i-1);
    end
end
final_x = lat(end);
final_y = long(end);
out(:,1) = lat;
out(:,2) = long;
out(:,3) = u(:, 3);

lat_out = out(:,1);
long_out = out(:, 2);
z_out =  out(:, 3);

== matlab function ModelForSlidesFeb/Environment & Data/Roadrunner Port/Pack Actor Pose/Pose Generation ==
  data: pose input; currPose output
function currPose = generatePose(pose)

yaw = deg2rad(pose(3));
rotm = eul2rotm([yaw 0 0]);

currPose = [[rotm [pose(1:2) 0]']; [0 0 0 1]];
% currPose = [[rotm [pose(1:2) 235]']; [0 0 0 1]];

== matlab function ModelForSlidesFeb/Environment & Data/Roadrunner Port/Pack Actor Pose/Velocity XYZ Components ==
  data: yaw input size=1; velocity output size=[1 3]; speed input size=1
function velocity = computeVelocity(yaw, speed)

% Output velocity vector (x,y,z)
velocity = speed * [-sind(yaw) cosd(yaw) 0];

== matlab function ModelForSlidesFeb/Environment & Data/Sensors & Perception/Tracking/MATLAB Function ==
  data: u input; y output; y1 output
function [y,y1] = fcn(u)
TracksNum = u.NumTracks;
y = zeros(20,1);
for k = 1:TracksNum
    y(k) = u.Tracks(k).ObjectAttributes.TargetIndex;
end
y1 = u.Tracks(1).ObjectAttributes.TargetIndex;

== matlab function ModelForSlidesFeb/Vehicle Dynamics/VehicleDynamics/MATLAB Function ==
  data: InitialPos input; Xo output; Yo output
function [Xo, Yo] = fcn(InitialPos)

Xo = InitialPos(1);
Yo = InitialPos(2);

== matlab function ModelForSlidesFeb/Environment & Data/Roadrunner Port/ENU to NWD/MATLAB Function2 ==
  data: u input; y output; y1 output
function [y,y1] = fcn(u)

y = u(:,1);
y1=u(:,2);

== matlab function ModelForSlidesFeb/Environment & Data/Roadrunner Port/ENU to NWD/2D RefWaypoints ==
  data: u input; y output
function y = fcn(u)

y = u(:,1:2);
end

== matlab function ModelForSlidesFeb/Behavioural Planner/MATLAB Function4 ==
  data: tracks input; y output; CurrentPose input; curr_vel input; tsim input; state input; g output; Te_e output; Te_l output; h output; entryTimes output; exitTimes output; entryPed output; exitPed output; entryProjected output; exitProjected output; vehicleoverlap output; pedestrianoverlap output; projectedoverlap output; Go input
function [y,g,Te_e,Te_l,h,entryTimes,exitTimes,entryPed,exitPed,entryProjected,exitProjected,vehicleoverlap,pedestrianoverlap,projectedoverlap] = UnprotectedLeftTurn(tracks,CurrentPose,curr_vel,tsim,state,Go)

if Go~=1
        y = -1;
        g = -1;
        Te_e = 0;
        Te_l = 0;
        h = -1 * ones(1, length(tracks.Actors));
        entryTimes = -1 * ones(1, length(tracks.Actors));
        exitTimes = -1 * ones(1, length(tracks.Actors));
        entryProjected = -1 * ones(1, length(tracks.Actors));
        exitProjected = -1 * ones(1, length(tracks.Actors));
        entryPed = -1 * ones(1, length(tracks.Actors));
        exitPed = -1 * ones(1, length(tracks.Actors));
        vehicleoverlap = false;
        pedestrianoverlap = false;
        projectedoverlap = false;
        return;  % Exit the function
 end






num_actors=length(tracks.Actors);
SL=15.6; % Speed Limit
y=-1;
g=-1;
t=-1;
h=-1*ones(1,num_actors);
Te_e=0;
Te_l=0;
EntryVc=0;
vehicleoverlap=false; %remove
pedestrianoverlap=false;
projectedoverlap=false;



    entryTimes =-1*ones(1,num_actors);
    
    exitTimes = -1*ones(1,num_actors);
    entryProjected=-1*ones(1,num_actors);
    exitProjected=-1*ones(1,num_actors);
    entryPed=-1*ones(1,num_actors);
    exitPed=-1*ones(1,num_actors);





if state==3 || state==4 || state ==5 || state ==1 % Either Green or Red/Yellow after Limit Line(Means we are already inside the intersection)[CHANGE CONDITION}
    if CurrentPose(1,1)<=-1 % && curr_vel>.50 % Means Ego is before the Limit Line
        Te_e=tsim+ abs(CurrentPose(1,1)-(-1))/4;              %curr_vel
        Te_l=tsim+ (sqrt((CurrentPose(1)-(14.920))^2+(CurrentPose(2)-15.28)^2))/4; %Time from current position to Limit Line on turning lane..(change distance to reflect curved distance)
        g=1;
       % Remove all g's later.. not needed
        
%     elseif CurrentPose(1,1)<-1 && curr_vel<=0.1 % Means Ego has stopped at/Before Limit Line
%         Te_e=tsim+ abs(CurrentPose(1,1)-(-1))/10;  %Assume that ego has some velocity, to calculate the window
%         Te_l=tsim+ (sqrt((CurrentPose(1)-(14.920))^2+(CurrentPose(2)-15.28)^2))/10; % Same as previous case
%         g=2;
    elseif CurrentPose(1,1)>-1 && curr_vel>0.1
        Te_e=tsim;
        Te_l=tsim+ (sqrt((CurrentPose(1)-(14.920))^2+(CurrentPose(2)-15.28)^2))/curr_vel;
        g=3;
    else
        Te_e=tsim;
        Te_l=tsim+ (sqrt((CurrentPose(1)-(14.920))^2+(CurrentPose(2)-15.28)^2))/4;
        g=4;
    end
    
    



    for i=1:num_actors
        if  tracks.Actors(i).ActorID > 7  % For vehicle actors
            if  -1*(tracks.Actors(i).Velocity(1)) < SL-0.5  % When Actor is below the speed limit(or between 9.5 and 10m/s)
                if (-0.85<=tracks.Actors(i).Position(1)) && (tracks.Actors(i).Position(1)<=23) % Actor is inside the Intersection, hence entry point is Tsim -0.85
               EntryVc= tsim; %Time for Actor to reach entry point
               ExitVc=tsim+((tracks.Actors(i).Position(1)-(-0.8))/(-1*(tracks.Actors(i).Velocity(1))));
               Entrys=tsim; %Time for Actor to reach entry point
               Exits=tsim+((tracks.Actors(i).Position(1)-(-0.8))/SL);% tIME for actor to reach exit point
               h(i)=1;
               entryTimes(i)=EntryVc;
               
               exitTimes(i)= ExitVc;
               entryProjected(i)=Entrys;
               exitProjected(i)=Exits;

                elseif tracks.Actors(i).Position(1)<-0.85  % Actor has exited the intersection, so we dont want to consider.. Hence arbitrary times: -0.85

               EntryVc= 0; %Time for Actor to reach entry point
               ExitVc=0;
               Entrys=0; %Time for Actor to reach entry point
               Exits=0;% tIME for actor to reach exit point

               entryTimes(i)=EntryVc;
               
               exitTimes(i)= ExitVc;
               entryProjected(i)=Entrys;
               exitProjected(i)=Exits;
               h(i)=0;
               


                else % This is the main case.. when actor is about to enter intersection
               EntryVc= tsim+((tracks.Actors(i).Position(1)-(26))/(-1*(tracks.Actors(i).Velocity(1)))); %Time for Actor to reach entry point
               ExitVc=tsim+((tracks.Actors(i).Position(1)-(-0.8))/(-1*(tracks.Actors(i).Velocity(1))));
               Entrys=tsim+ ((tracks.Actors(i).Position(1)-(26))/SL); %Time for Actor to reach entry point
               Exits=tsim+ ((tracks.Actors(i).Position(1)-(-0.8))/SL);% tIME for actor to reach exit point
               h(i)=2;
               

               entryTimes(i)=EntryVc;
               
               exitTimes(i)= ExitVc;
               entryProjected(i)=Entrys;
               exitProjected(i)=Exits;

                end
            else % When actor at speed limit
                if (-0.85<=tracks.Actors(i).Position(1)) && (tracks.Actors(i).Position(1)<=23) % Same cases as above
                EntryVc=tsim; %Time for Actor to reach entry point
                ExitVc=tsim+ ((tracks.Actors(i).Position(1)-(-0.8))/SL);
                entryTimes(i)=EntryVc;
                
                exitTimes(i)= ExitVc;
                h(i)=3;
                

                elseif tracks.Actors(i).Position(1)<-0.85  %Same cases as above -0.85
                EntryVc=0; %Time for Actor to reach entry point
                ExitVc=0;
                entryTimes(i)=EntryVc;
                %exit(i)=ExitVc;
                exitTimes(i)= ExitVc;
                h(i)=4;
                


                else %Same cases as above

                EntryVc=tsim+ ((tracks.Actors(i).Position(1)-(26))/SL); %Time for Actor to reach entry point
                ExitVc=tsim+ ((tracks.Actors(i).Position(1)-(-0.8))/SL);
                entryTimes(i)=EntryVc;
                
                exitTimes(i)= ExitVc;
                h(i)=5;
               




                end


            end

        elseif (6< tracks.Actors(i).ActorID) && (tracks.Actors(i).ActorID <8)%For pedestrians, will change based on number of pedestrians    
            if tracks.Actors(i).Position(1) > 16.5
             EntryP= tsim+((tracks.Actors(i).Position(1)-(16.5))/(-1*(tracks.Actors(i).Velocity(1))));
             %EntryP= tsim+(tracks.Actors(i).Position(2)-(-45)/(-1*tracks.Actors(i).Velocity(2))); %Time for Actor to reach entry point
             %ExitP=tsim+(tracks.Actors(i).Position(2)-(-50)/(-1*tracks.Actors(i).Velocity(2)));
             ExitP= tsim+((tracks.Actors(i).Position(1)-(13.1))/(-1*(tracks.Actors(i).Velocity(1))));

            elseif tracks.Actors(i).Position(1) < 16.5 && tracks.Actors(i).Position(1) >13.1
                 EntryP=tsim;
                 ExitP= tsim+((tracks.Actors(i).Position(1)-(13.1))/(-1*(tracks.Actors(i).Velocity(1))));

            else
                EntryP=-1;
                ExitP=-1;
%             else
%              %Time for Actor to reach entry point
%              EntryP= tsim+((tracks.Actors(i).Position(2)-(13.1))/(-1*(tracks.Actors(i).Velocity(1))));
%              ExitP= tsim+((tracks.Actors(i).Position(2)-(16.5))/(-1*(tracks.Actors(i).Velocity(1))));
             
            end
            entryPed(i)=EntryP;
            exitPed(i)= ExitP;
        end

    end




    % Check for overlap between Ego Times and Actor Times

vehicleoverlap = false;
pedestrianoverlap = false;
projectedoverlap = false;

for i = 1:length(entryTimes)
    if Te_e <= exitTimes(i) && Te_l >= entryTimes(i)
        vehicleoverlap = true;
        y = 0; % Stay
        break;
    end
end

if ~vehicleoverlap
    for i = 1:length(entryPed)
        if Te_e <= exitPed(i) && Te_l >= entryPed(i)
            pedestrianoverlap = true;
            y = 0; % Stay
            break;
        end
    end
end

if ~vehicleoverlap && ~pedestrianoverlap
    for i = 1:length(entryProjected)
        if Te_e <= exitProjected(i) && Te_l >= entryProjected(i)
            projectedoverlap = true;
            y = 1; % Go to the next point
            break;
        end
    end
end

if ~vehicleoverlap && ~pedestrianoverlap && ~projectedoverlap
    y = 2; % Set y to 2 only if none of the conditions are met
end

















            


end

== matlab function ModelForSlidesFeb/Controllers/Subsystem2/MATLAB Function ==
  data: u input; accel output; decel output
function [accel, decel] = fcn(u)
if(u>0)
    accel=u; decel=0;
elseif(u<0)
    accel=0; decel=-u;
else
    accel=0;decel=0;
end

== matlab function ModelForSlidesFeb/Controllers/Subsystem2/Subsystem/Desired Velocity Profile ==
  data: MaxBrakeFlag output; CurrVel input; DesiredDecel output; RelDist input; Dist1 output; StoppingDist input
function [MaxBrakeFlag,DesiredDecel,Dist1] = VelocityProfile(CurrVel,RelDist,StoppingDist)
% time remaining = (current velocity) / (deceleration).
% desired velocity = (stopping distance - current distance) / time remaining.
Dist1 = RelDist - (2.6850+1);
Dist = Dist1 - StoppingDist;
if Dist1 <= 2
    MaxBrakeFlag = 1;
    DesiredDecel = 0;
else
    MaxBrakeFlag = 0;
    DesiredDecel = min((CurrVel^2)/(2*Dist),3.5);
end
%     Dist = RelDist - (2.6850 + 3);
%     Decel = (CurrVel^2)/(2*Dist);
%     RemainingTime = CurrVel/Decel;
%     DesiredVel = Dist/RemainingTime; % DesiredVel = CurrVel/2

== matlab function ModelForSlidesFeb/Controllers/Subsystem2/Subsystem/Function-Call Subsystem/MATLAB Function1 ==
  data: Vel input; BrakingAcc output; RelDist input
function BrakingAcc = fcn(Vel,RelDist)

DistOffset = 1;
Dist = RelDist - DistOffset;
BrakingAcc = (Vel^2)/(2*Dist);
